simulink library "martin_sean_RoombaLib"  (R2017a)
settings: Solver=VariableStepAuto  StartTime=0.0  StopTime=10.0  RelTol=1e-3
settings Model: Creator=tuf53749  LastModifiedBy=Sean

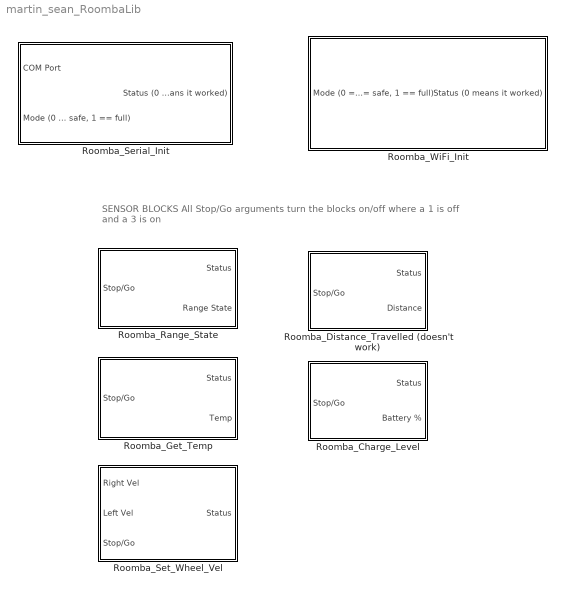
== system martin_sean_RoombaLib ==
  note: SENSOR BLOCKS
      |
      | All Stop/Go arguments turn the blocks on/off where a 1 is off and a 3 is on
  Roomba_Charge_Level : Subsystem  Description=Returns the battery charge level on the Roomba as a percentage. Updates every 100 seconds.  mask(Charge Level Roomba){}
      mask help: Returns the battery charge level on the Roomba as a percentage. Updates every 100 seconds.
  Roomba_Distance_Travelled (doesn't work) : Subsystem  mask(Distance Travelled Roomba){}
      mask help: Takes in the counts from the Roomba's wheel encoders. Using the diameter of the wheels this value is manipulated to obtain a distance the wheels have spun. STILL NEEDS TO BE FINISHED.
  Roomba_Get_Temp : Subsystem  Description=|  mask(Get Temperature Roomba){}
      | Returns the value of the temperature sensor on the Roomba in degrees Celcius. Updates every
      | 30 seconds.
      mask help: Returns the value of the temperature sensor on the Roomba in degrees Celcius. Updates every 30 seconds.
  Roomba_Range_State : Subsystem  Description=|  mask(Range State Roomba){}
      | Returns [1x6] array containing the state of the six IR sensors on the front of the Roomba. A 
      | '1' indicates there is an object ahead and a '0' indicates no object.
      mask help:
      | Returns [1x6] array containing the state of the six IR sensors on the front of the Roomba. A
      | '1' indicates there is an object ahead and a '0' indicates no object.
  Roomba_Serial_Init : Subsystem  Description=|  Priority=-1000  StartFcn=|  StopFcn=|  mask(Roomba Serial Port Initialization){}
      Description=|
      | Initializes a serial connection to the Roomba. Takes the COM Port number and mode as inputs.
      | For instance, COM Port = 3 and Mode = 1 will set up a connection to the Roomba on COM3
      | and place it in 'full' mode.
      | 
      | A 0 is returned after successful initialization.
      StartFcn=|
      | %clear the workspace of old Roomba obj
      | clear all;
      StopFcn=|
      | %this sends a reset and stop cmd to the 
      | %Roomba before quiting sim
      | coder.extrinsic('RoombaClose');
      | RoombaClose;
      mask help:
      | Initializes a serial connection to the Roomba. Takes the COM Port number and mode as inputs.
      | For instance, COM Port = 3 and Mode = 1 will set up a connection to the Roomba on COM3
      | and place it in 'full' mode.
      |
      | A 0 is returned after successful initialization.
  Roomba_Set_Wheel_Vel : Subsystem  Description=|  mask(Set Wheel Velocity Roomba){}
      | Sets the right and left wheel velocities on the Roomba. The values are in meters/sec between 
      | [-0.5, 0.5]. Negative velocity is backwards.
      mask help: Sets the right and left wheel velocities on the Roomba. The values are in meters/sec between [-0.5, 0.5]. Negative velocity is backwards.
  Roomba_WiFi_Init : Subsystem  Description=|  Priority=-1000  StartFcn=|  StopFcn=|  mask(Roomba WiFi Initialization){}
      Description=|
      | Initializes a WiFi connection to the Roomba. The RooWiFi module is used. Takes the mode as an
      | input. For instance, Mode = 1 will set up a connection to the Roomba over RooWiFi on 10.0.0.1
      | and place it in 'full' mode.
      | 
      | A 0 is returned after successful initialization.
      | 
      | RooWiFi documentation:
      | http://www.roowifi.com/wp-content/uploads/RwRemote_User_Guide_v2_rev15.pdf
      StartFcn=|
      | %clear the workspace of old Roomba obj
      | clear all;
      StopFcn=|
      | %this sends a reset and stop cmd to the 
      | %Roomba before quiting sim
      | coder.extrinsic('RoombaClose');
      | RoombaClose;
      mask help:
      | Initializes a WiFi connection to the Roomba. The RooWiFi module is used. Takes the mode as an
      | input. For instance, Mode = 1 will set up a connection to the Roomba over RooWiFi on 10.0.0.1
      | and place it in 'full' mode.
      |
      | A 0 is returned after successful initialization.
      |
      | RooWiFi documentation:
      | http://www.roowifi.com/wp-content/uploads/RwRemote_User_Guide_v2_rev15.pdf

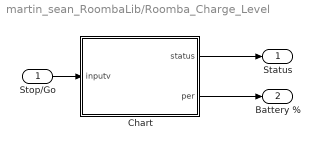
== system martin_sean_RoombaLib/Roomba_Charge_Level ==
  Stop/Go : Inport
  Chart : Stateflow chart  TreatAsAtomicUnit=on
  Status : Outport
  Battery % : Outport  Port=2
  wires:
  Stop/Go/1 -> Chart/1(inputv)
  Chart/1(status) -> Status/1
  Chart/2(per) -> Battery %/1

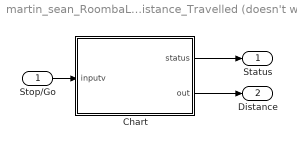
== system martin_sean_RoombaLib/Roomba_Distance_Travelled (doesn't work) ==
  Stop/Go : Inport
  Chart : Stateflow chart  TreatAsAtomicUnit=on
  Status : Outport
  Distance : Outport  Port=2
  wires:
  Chart/2(out) -> Distance/1
  Stop/Go/1 -> Chart/1(inputv)
  Chart/1(status) -> Status/1

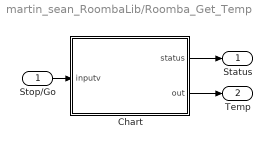
== system martin_sean_RoombaLib/Roomba_Get_Temp ==
  Stop/Go : Inport
  Chart : Stateflow chart  TreatAsAtomicUnit=on
  Status : Outport
  Temp : Outport  Port=2
  wires:
  Stop/Go/1 -> Chart/1(inputv)
  Chart/1(status) -> Status/1
  Chart/2(out) -> Temp/1

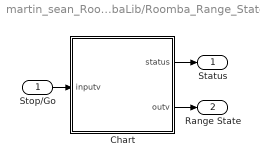
== system martin_sean_RoombaLib/Roomba_Range_State ==
  Stop/Go : Inport
  Chart : Stateflow chart  TreatAsAtomicUnit=on
  Status : Outport
  Range State : Outport  Port=2
  wires:
  Chart/1(status) -> Status/1
  Chart/2(outv) -> Range State/1
  Stop/Go/1 -> Chart/1(inputv)

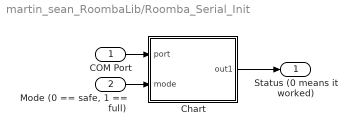
== system martin_sean_RoombaLib/Roomba_Serial_Init ==
  COM Port : Inport
  "Mode (0 == safe, 1 == full)" : Inport  Port=2
  Chart : Stateflow chart  TreatAsAtomicUnit=on
  Status (0 means it worked) : Outport
  wires:
  COM Port/1 -> Chart/1(port)
  "Mode (0 == safe, 1 == full)"/1 -> Chart/2(mode)
  Chart/1(out1) -> Status (0 means it worked)/1

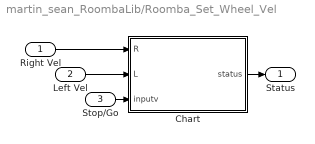
== system martin_sean_RoombaLib/Roomba_Set_Wheel_Vel ==
  Right Vel : Inport  OutMin=[-0.5]  OutMax=[0.5]
  Left Vel : Inport  Port=2  OutMin=[-0.5]  OutMax=[0.5]
  Stop/Go : Inport  Port=3
  Chart : Stateflow chart  TreatAsAtomicUnit=on
  Status : Outport
  wires:
  Right Vel/1 -> Chart/1(R)
  Left Vel/1 -> Chart/2(L)
  Chart/1(status) -> Status/1
  Stop/Go/1 -> Chart/3(inputv)

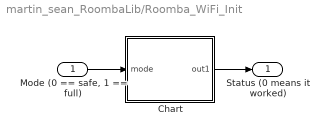
== system martin_sean_RoombaLib/Roomba_WiFi_Init ==
  "Mode (0 == safe, 1 == full)" : Inport
  Chart : Stateflow chart  TreatAsAtomicUnit=on
  Status (0 means it worked) : Outport
  wires:
  "Mode (0 == safe, 1 == full)"/1 -> Chart/1(mode)
  Chart/1(out1) -> Status (0 means it worked)/1

== stateflow chart martin_sean_RoombaLib/Roomba_Range_State/Chart ==
  state Init_Vector
    en:
    outv = [0,0,0,0,0,0];
    status=0;
  state Limbo
    en,du:
    outv=RangeStateRoomba_Get;
    status=2;
  state NoCommand
    en:
    outv = [0,0,0,0,0,0];
    status=1;
  (default) -> Init_Vector
  Init_Vector -> NoCommand : after(0.1,sec)
  NoCommand -> Limbo : [inputv==3]
  Limbo -> Limbo [order 2] : after(0.1,sec)
  Limbo -> NoCommand [order 1] : [inputv==1]
  data: y function_output; status output; outv output; inputv input
  function y = RangeStateRoomba_Get:
    | function y = RangeStateRoomba_Get
    | persistent obj
    | y = [0,0,0,0,0,0];
    | coder.extrinsic('RangeStateRoomba');
    | coder.extrinsic('evalin');
    | coder.extrinsic('get');
    | if isempty(obj)
    |     obj = evalin('base','objWs');
    | end
    | y = RangeStateRoomba(obj);

== stateflow chart martin_sean_RoombaLib/Roomba_Set_Wheel_Vel/Chart ==
  state StoppedWheels
    en:
    SetWheelVelRoomba_Get(0,0);
    status=0;
  state Limbo
    en:
    SetWheelVelRoomba_Get(R,L);
    status=1;
  (default) -> StoppedWheels
  Limbo -> StoppedWheels [order 1] : [inputv==1]
  StoppedWheels -> Limbo : [inputv==3]
  Limbo -> Limbo [order 2] : after(0.1,sec)
  data: right function_input [-0.5..0.5]; left function_input [-0.5..0.5]; status output; R input [-0.5..0.5]; L input [-0.5..0.5]; inputv input
  function SetWheelVelRoomba_Get(right,left):
    | function SetWheelVelRoomba_Get(right,left)
    | persistent obj
    | coder.extrinsic('SetWheelVelRoomba');
    | coder.extrinsic('evalin');
    | coder.extrinsic('get');
    | if isempty(obj)
    |     obj = evalin('base','objWs');
    | end
    | y = SetWheelVelRoomba(obj,right,left);

== stateflow chart martin_sean_RoombaLib/Roomba_Serial_Init/Chart ==
  state State
    en,du:
    serial_Init(port,mode);
    out1 = 0;
  (default) -> State
  data: x function_input; y function_input; port input; out1 output; mode input
  function serial_Init(x,y):
    | function serial_Init(x,y)
    | coder.extrinsic('RoombaInit');
    | coder.extrinsic('num2str');
    | coder.extrinsic('strcat');
    | coder.extrinsic('instrreset');
    | coder.extrinsic('instrfind');
    | coder.extrinsic('delete');
    | coder.extrinsic('serial');
    | coder.extrinsic('assignin');
    | persistent obj
    | mode_string = 'safe';
    | if isempty(obj)
    |     if y == 1
    |         mode_string = 'full';
    |     end
    |     obj=RoombaInit(x,mode_string);
    |     assignin('base','objWs',obj);
    | end

== stateflow chart martin_sean_RoombaLib/Roomba_WiFi_Init/Chart ==
  state State
    en,du:
    wifi_Init(mode);
    out1 = 0;
  (default) -> State
  data: y function_input; out1 output; mode input
  function wifi_Init(y):
    | function wifi_Init(y)
    | coder.extrinsic('RoombaInit_tcp');
    | coder.extrinsic('num2str');
    | coder.extrinsic('strcat');
    | coder.extrinsic('instrreset');
    | coder.extrinsic('instrfind');
    | coder.extrinsic('delete');
    | coder.extrinsic('serial');
    | coder.extrinsic('assignin');
    | persistent obj
    | mode_string = 'safe';
    | if isempty(obj)
    |     if y == 1
    |         mode_string = 'full';
    |     end
    |     obj=RoombaInit_tcp('10.0.0.1',mode_string);
    |     assignin('base','objWs',obj);
    | end

== stateflow chart martin_sean_RoombaLib/Roomba_Get_Temp/Chart ==
  state StoppedWheels
    en:
    out = nan;
    status=0;
  state Limbo
    en:
    out = RoombaTemperature_Get;
    status=1;
  (default) -> StoppedWheels
  Limbo -> StoppedWheels [order 1] : [inputv==1]
  StoppedWheels -> Limbo : [inputv==3]
  Limbo -> Limbo [order 2] : after(30,sec)
  data: y function_output; status output; inputv input; out output
  function y = RoombaTemperature_Get:
    | function y = RoombaTemperature_Get
    | persistent obj
    | coder.extrinsic('TemperatureRoomba');
    | coder.extrinsic('evalin');
    | coder.extrinsic('get');
    | if isempty(obj)
    |     obj = evalin('base','objWs');
    | end
    | y = TemperatureRoomba(obj);

== stateflow chart martin_sean_RoombaLib/Roomba_Distance_Travelled (doesn't work)/Chart ==
  state ResetStart
    en:
    out = 0;
    status=0;
  state Limbo
    en:
    counts = EncoderSensorsRoomba_Get;
    out = counts*pi*2*0.036/508.8;
    status=1;
  (default) -> ResetStart
  Limbo -> ResetStart [order 1] : [inputv==1]
  ResetStart -> Limbo : [inputv==3]
  Limbo -> Limbo [order 2] : after(0.1,sec)
  data: y function_output; status output; inputv input; out output; counts local
  function y = EncoderSensorsRoomba_Get:
    | function y = EncoderSensorsRoomba_Get
    | persistent obj
    | coder.extrinsic('TemperatureRoomba');
    | coder.extrinsic('evalin');
    | coder.extrinsic('get');
    | if isempty(obj)
    |     obj = evalin('base','objWs');
    | end
    | y = TemperatureRoomba(obj);

== stateflow chart martin_sean_RoombaLib/Roomba_Charge_Level/Chart ==
  state ResetStart
    en:
    per = nan;
    status=0;
  state Limbo
    en:
    [charge,cap,per] = BatteryChargeReaderRoomba_Get;
    status=1;
  (default) -> ResetStart
  ResetStart -> Limbo : [inputv==3]
  Limbo -> ResetStart [order 1] : [inputv==1]
  Limbo -> Limbo [order 2] : after(100,sec)
  data: x function_output; y function_output; z function_output; status output; inputv input; charge local; per output; cap local
  function [x,y,z] = BatteryChargeReaderRoomba_Get:
    | function [x,y,z] = BatteryChargeReaderRoomba_Get
    | persistent obj
    | coder.extrinsic('BatteryChargeReaderRoomba');
    | coder.extrinsic('evalin');
    | coder.extrinsic('get');
    | if isempty(obj)
    |     obj = evalin('base','objWs');
    | end
    | [x,y,z] = BatteryChargeReaderRoomba(obj);
